simulink model "RadioReceiver_FP_clean_PIPELINED_64bit"  (R2017a)
settings: Solver=FixedStepDiscrete  StartTime=0.0  StopTime=10.0  RelTol=1e-3
InitFcn:
  | barker = comm.BarkerCode('SamplesPerFrame', 28, 'Length', 11);
  | seq = barker()+1;
  | M = 4;
  | hPSKModTrain   = comm.PSKModulator(M, ...
  |     'PhaseOffset',pi/4, ...
  |     'SymbolMapping','Binary');
  | xPreambleSeq = hPSKModTrain(seq);
  | 
  | 
  | %%%%%%%%%%%%
  | 
  | % AGC Preamble
  | reps = 5;
  | barker = comm.BarkerCode('SamplesPerFrame', 16, 'Length', 13);
  | seq = barker()+1;
  | %preamble = zeros(16*reps,1);
  | preambleFull = repmat(seq,reps,1);
  | rctFilt = comm.RaisedCosineTransmitFilter('FilterSpanInSymbols', 128,...
  | 'RolloffFactor',0.5,...
  | 'OutputSamplesPerSymbol',4);
  | preambleFullFilt = rctFilt(preambleFull);
  | 
  | %%%%%%%%%%%%
  | 
  | RadioSampleRate = 1e6;
  | %RadioSampleRate = 20e6;
  | RadioFrameLength = 1e5;
  | 
  | VibertiTracebackLength = 34+20;
  | numTrainingSamples = 250;
  | crc32Poly = [1 0 0 0 0 0 1 0 0 1 1 0 0 0 0 0 1 0 0 0 1 1 1 0 1 1 0 1 1 0 1 1 1];
  | crcDecodeLag = length(crc32Poly)-1+2;
  | 
  | %%%%%%%%%%%%
  | 
  | beta = 0.5;
  | span = 8;
  | sps = 4;
  | filterGain = 1;
  | coeff = rcosdesign(beta, span, sps, 'sqrt')*filterGain;
  | 
  | %%%%%%%%%%%%
  | 
  | samplesPerSymbol = 4;
  | maxPacketBits = 8*1500;
  | bItsPerSymbol = 2;
  | CodeRate = 2;
  | tailSymbols = 40;
  | maxPayloadSymbols = maxPacketBits*CodeRate/bItsPerSymbol+tailSymbols;
undefined symbols (not defined in the file or in its folder): j
libraries: dsphdlfiltering x20, simulink x15, dspstat3 x2, hdlsllib x2, commdigbbndpm3 x2, commsource2 x1, commcrc2 x1, commcnvcod2 x1, commseqgen3 x1, commutil2 x1
(part 2 of 2)

== system RadioReceiver_FP_clean_PIPELINED_64bit/Receiver HDL/Frame Recover/Barker Locate/Measure Phase Ambiguity1/Find Max and Set Output Shift ==
  In1 : Inport
  In2 : Inport  Port=2
  In4 : Inport  Port=3
  In5 : Inport  Port=4
  Enable : EnablePort
  Complex to Real-Imag{,1..3} (4 alike) : ComplexToRealImag  Output=Imag
  Direct Lookup Table (n-D) : LookupNDDirect  NumberOfTableDimensions=1  Table=exp(-(0:pi/2:(pi*3/2)) .* 1i).'  DiagnosticForOutOfRangeInput=Error  TableDataTypeStr=fixdt(1,16,13)
  Display : Display
  Display1 : Display
  Maximum : dspstat3/Maximum  operation=maximum  fcn=Index  indexBase=Zero  operateOver=Each column  Dimension=1  InputProcessing=Columns as channels (frame based)  reset=None  roiEnable=off  roiType=Rectangles  roiPortion=Entire ROI  roiOutput=Individual statistics for each ROI  roiFlag=off  roundingMode=Floor  overflowMode=off  accumDataTypeStr=Inherit: Same as product output  accumLastDataTypeStr=Inherit: Same as product output
  Vector Concatenate : Concatenate  NumInputs=4
  Vector Concatenate1 : Concatenate  NumInputs=4
  Out1 : Outport  InitialOutput=0
  wires:
  Direct Lookup Table (n-D)/1 -> Out1/1
  In4/1 -> Vector Concatenate1/3, Complex to Real-Imag2/1
  In2/1 -> Vector Concatenate1/2, Complex to Real-Imag1/1
  In5/1 -> Vector Concatenate1/4, Complex to Real-Imag3/1
  In1/1 -> Vector Concatenate1/1, Complex to Real-Imag/1
  Maximum/1 -> Direct Lookup Table (n-D)/1
  Vector Concatenate/1 -> Display/1, Maximum/1
  Vector Concatenate1/1 -> Display1/1
  Complex to Real-Imag1/1 -> Vector Concatenate/2
  Complex to Real-Imag3/1 -> Vector Concatenate/4
  Complex to Real-Imag2/1 -> Vector Concatenate/3
  Complex to Real-Imag/1 -> Vector Concatenate/1

== system RadioReceiver_FP_clean_PIPELINED_64bit/Receiver HDL/Frame Recover/Barker Locate/Measure Phase Ambiguity1/HDL Opt Complex FIR4 ==
  In1 : Inport
  validIn : Inport  Port=2
  Add : Sum  Inputs=+-  AccumDataTypeStr=fixdt(1,16,0)
  Complex to Real-Imag : ComplexToRealImag
  Discrete FIR Filter HDL Optimized : dsphdlfiltering/Discrete FIR Filter HDL Optimized  Numerator=real(Taps)  Sharing=off  SharingFactor=2  SimulateUsing=Code generation  roundingMode=Floor  overflowMode=off  CoefficientsDataTypeStr=Inherit: Same word length as input  CoefficientsMin=[]  CoefficientsMax=[]  OutputDataTypeStr=fixdt(1,16,0)  OutputMin=[]  OutputMax=[]  ValidInPort=on  ReadyPort=off
      settings: SourceProductName=DSP System Toolbox  SourceProductBaseCode=DS
  Discrete FIR Filter HDL Optimized1 : dsphdlfiltering/Discrete FIR Filter HDL Optimized  Numerator=imag(Taps)  Sharing=off  SharingFactor=2  SimulateUsing=Code generation  roundingMode=Floor  overflowMode=off  CoefficientsDataTypeStr=Inherit: Same word length as input  CoefficientsMin=[]  CoefficientsMax=[]  OutputDataTypeStr=fixdt(1,16,0)  OutputMin=[]  OutputMax=[]  ValidInPort=on  ReadyPort=off
      settings: SourceProductName=DSP System Toolbox  SourceProductBaseCode=DS
  Discrete FIR Filter HDL Optimized2 : dsphdlfiltering/Discrete FIR Filter HDL Optimized  Numerator=real(Taps)  Sharing=off  SharingFactor=2  SimulateUsing=Code generation  roundingMode=Floor  overflowMode=off  CoefficientsDataTypeStr=Inherit: Same word length as input  CoefficientsMin=[]  CoefficientsMax=[]  OutputDataTypeStr=fixdt(1,16,0)  OutputMin=[]  OutputMax=[]  ValidInPort=on  ReadyPort=off
      settings: SourceProductName=DSP System Toolbox  SourceProductBaseCode=DS
  Discrete FIR Filter HDL Optimized3 : dsphdlfiltering/Discrete FIR Filter HDL Optimized  Numerator=imag(Taps)  Sharing=off  SharingFactor=2  SimulateUsing=Code generation  roundingMode=Floor  overflowMode=off  CoefficientsDataTypeStr=Inherit: Same word length as input  CoefficientsMin=[]  CoefficientsMax=[]  OutputDataTypeStr=fixdt(1,16,0)  OutputMin=[]  OutputMax=[]  ValidInPort=on  ReadyPort=off
      settings: SourceProductName=DSP System Toolbox  SourceProductBaseCode=DS
  Logical Operator : Logic  Inputs=4  AllPortsSameDT=off  OutDataTypeStr=boolean
  Real-Imag to Complex : RealImagToComplex
  Subtract : Sum  OutDataTypeStr=int16
  Out1 : Outport
  validOut : Outport  Port=2
  wires:
  Discrete FIR Filter HDL Optimized/1 -> Add/1
  Logical Operator/1 -> validOut/1
  Discrete FIR Filter HDL Optimized/2 -> Logical Operator/1
  Discrete FIR Filter HDL Optimized1/2 -> Logical Operator/2
  Discrete FIR Filter HDL Optimized1/1 -> Add/2
  validIn/1 -> Discrete FIR Filter HDL Optimized3/2, Discrete FIR Filter HDL Optimized2/2, Discrete FIR Filter HDL Optimized1/2, Discrete FIR Filter HDL Optimized/2
  In1/1 -> Complex to Real-Imag/1
  Complex to Real-Imag/1 -> Discrete FIR Filter HDL Optimized3/1, Discrete FIR Filter HDL Optimized/1
  Discrete FIR Filter HDL Optimized2/2 -> Logical Operator/3
  Discrete FIR Filter HDL Optimized3/2 -> Logical Operator/4
  Complex to Real-Imag/2 -> Discrete FIR Filter HDL Optimized2/1, Discrete FIR Filter HDL Optimized1/1
  Discrete FIR Filter HDL Optimized2/1 -> Subtract/1
  Discrete FIR Filter HDL Optimized3/1 -> Subtract/2
  Real-Imag to Complex/1 -> Out1/1
  Subtract/1 -> Real-Imag to Complex/2
  Add/1 -> Real-Imag to Complex/1

== system RadioReceiver_FP_clean_PIPELINED_64bit/Receiver HDL/Frame Recover/Barker Locate/Measure Phase Ambiguity1/HDL Opt Complex FIR5 ==
  In1 : Inport
  validIn : Inport  Port=2
  Add : Sum  Inputs=+-  AccumDataTypeStr=fixdt(1,16,0)
  Complex to Real-Imag : ComplexToRealImag
  Discrete FIR Filter HDL Optimized : dsphdlfiltering/Discrete FIR Filter HDL Optimized  Numerator=real(Taps)  Sharing=off  SharingFactor=2  SimulateUsing=Code generation  roundingMode=Floor  overflowMode=off  CoefficientsDataTypeStr=Inherit: Same word length as input  CoefficientsMin=[]  CoefficientsMax=[]  OutputDataTypeStr=fixdt(1,16,0)  OutputMin=[]  OutputMax=[]  ValidInPort=on  ReadyPort=off
      settings: SourceProductName=DSP System Toolbox  SourceProductBaseCode=DS
  Discrete FIR Filter HDL Optimized1 : dsphdlfiltering/Discrete FIR Filter HDL Optimized  Numerator=imag(Taps)  Sharing=off  SharingFactor=2  SimulateUsing=Code generation  roundingMode=Floor  overflowMode=off  CoefficientsDataTypeStr=Inherit: Same word length as input  CoefficientsMin=[]  CoefficientsMax=[]  OutputDataTypeStr=fixdt(1,16,0)  OutputMin=[]  OutputMax=[]  ValidInPort=on  ReadyPort=off
      settings: SourceProductName=DSP System Toolbox  SourceProductBaseCode=DS
  Discrete FIR Filter HDL Optimized2 : dsphdlfiltering/Discrete FIR Filter HDL Optimized  Numerator=real(Taps)  Sharing=off  SharingFactor=2  SimulateUsing=Code generation  roundingMode=Floor  overflowMode=off  CoefficientsDataTypeStr=Inherit: Same word length as input  CoefficientsMin=[]  CoefficientsMax=[]  OutputDataTypeStr=fixdt(1,16,0)  OutputMin=[]  OutputMax=[]  ValidInPort=on  ReadyPort=off
      settings: SourceProductName=DSP System Toolbox  SourceProductBaseCode=DS
  Discrete FIR Filter HDL Optimized3 : dsphdlfiltering/Discrete FIR Filter HDL Optimized  Numerator=imag(Taps)  Sharing=off  SharingFactor=2  SimulateUsing=Code generation  roundingMode=Floor  overflowMode=off  CoefficientsDataTypeStr=Inherit: Same word length as input  CoefficientsMin=[]  CoefficientsMax=[]  OutputDataTypeStr=fixdt(1,16,0)  OutputMin=[]  OutputMax=[]  ValidInPort=on  ReadyPort=off
      settings: SourceProductName=DSP System Toolbox  SourceProductBaseCode=DS
  Logical Operator : Logic  Inputs=4  AllPortsSameDT=off  OutDataTypeStr=boolean
  Real-Imag to Complex : RealImagToComplex
  Subtract : Sum  OutDataTypeStr=int16
  Out1 : Outport
  validOut : Outport  Port=2
  wires:
  Discrete FIR Filter HDL Optimized/1 -> Add/1
  Logical Operator/1 -> validOut/1
  Discrete FIR Filter HDL Optimized/2 -> Logical Operator/1
  Discrete FIR Filter HDL Optimized1/2 -> Logical Operator/2
  Discrete FIR Filter HDL Optimized1/1 -> Add/2
  validIn/1 -> Discrete FIR Filter HDL Optimized3/2, Discrete FIR Filter HDL Optimized2/2, Discrete FIR Filter HDL Optimized1/2, Discrete FIR Filter HDL Optimized/2
  In1/1 -> Complex to Real-Imag/1
  Complex to Real-Imag/1 -> Discrete FIR Filter HDL Optimized3/1, Discrete FIR Filter HDL Optimized/1
  Discrete FIR Filter HDL Optimized2/2 -> Logical Operator/3
  Discrete FIR Filter HDL Optimized3/2 -> Logical Operator/4
  Complex to Real-Imag/2 -> Discrete FIR Filter HDL Optimized2/1, Discrete FIR Filter HDL Optimized1/1
  Discrete FIR Filter HDL Optimized2/1 -> Subtract/1
  Discrete FIR Filter HDL Optimized3/1 -> Subtract/2
  Real-Imag to Complex/1 -> Out1/1
  Subtract/1 -> Real-Imag to Complex/2
  Add/1 -> Real-Imag to Complex/1

== system RadioReceiver_FP_clean_PIPELINED_64bit/Receiver HDL/Frame Recover/Barker Locate/Measure Phase Ambiguity1/HDL Opt Complex FIR6 ==
  In1 : Inport
  validIn : Inport  Port=2
  Add : Sum  Inputs=+-  AccumDataTypeStr=fixdt(1,16,0)
  Complex to Real-Imag : ComplexToRealImag
  Discrete FIR Filter HDL Optimized : dsphdlfiltering/Discrete FIR Filter HDL Optimized  Numerator=real(Taps)  Sharing=off  SharingFactor=2  SimulateUsing=Code generation  roundingMode=Floor  overflowMode=off  CoefficientsDataTypeStr=Inherit: Same word length as input  CoefficientsMin=[]  CoefficientsMax=[]  OutputDataTypeStr=fixdt(1,16,0)  OutputMin=[]  OutputMax=[]  ValidInPort=on  ReadyPort=off
      settings: SourceProductName=DSP System Toolbox  SourceProductBaseCode=DS
  Discrete FIR Filter HDL Optimized1 : dsphdlfiltering/Discrete FIR Filter HDL Optimized  Numerator=imag(Taps)  Sharing=off  SharingFactor=2  SimulateUsing=Code generation  roundingMode=Floor  overflowMode=off  CoefficientsDataTypeStr=Inherit: Same word length as input  CoefficientsMin=[]  CoefficientsMax=[]  OutputDataTypeStr=fixdt(1,16,0)  OutputMin=[]  OutputMax=[]  ValidInPort=on  ReadyPort=off
      settings: SourceProductName=DSP System Toolbox  SourceProductBaseCode=DS
  Discrete FIR Filter HDL Optimized2 : dsphdlfiltering/Discrete FIR Filter HDL Optimized  Numerator=real(Taps)  Sharing=off  SharingFactor=2  SimulateUsing=Code generation  roundingMode=Floor  overflowMode=off  CoefficientsDataTypeStr=Inherit: Same word length as input  CoefficientsMin=[]  CoefficientsMax=[]  OutputDataTypeStr=fixdt(1,16,0)  OutputMin=[]  OutputMax=[]  ValidInPort=on  ReadyPort=off
      settings: SourceProductName=DSP System Toolbox  SourceProductBaseCode=DS
  Discrete FIR Filter HDL Optimized3 : dsphdlfiltering/Discrete FIR Filter HDL Optimized  Numerator=imag(Taps)  Sharing=off  SharingFactor=2  SimulateUsing=Code generation  roundingMode=Floor  overflowMode=off  CoefficientsDataTypeStr=Inherit: Same word length as input  CoefficientsMin=[]  CoefficientsMax=[]  OutputDataTypeStr=fixdt(1,16,0)  OutputMin=[]  OutputMax=[]  ValidInPort=on  ReadyPort=off
      settings: SourceProductName=DSP System Toolbox  SourceProductBaseCode=DS
  Logical Operator : Logic  Inputs=4  AllPortsSameDT=off  OutDataTypeStr=boolean
  Real-Imag to Complex : RealImagToComplex
  Subtract : Sum  OutDataTypeStr=int16
  Out1 : Outport
  validOut : Outport  Port=2
  wires:
  Discrete FIR Filter HDL Optimized/1 -> Add/1
  Logical Operator/1 -> validOut/1
  Discrete FIR Filter HDL Optimized/2 -> Logical Operator/1
  Discrete FIR Filter HDL Optimized1/2 -> Logical Operator/2
  Discrete FIR Filter HDL Optimized1/1 -> Add/2
  validIn/1 -> Discrete FIR Filter HDL Optimized3/2, Discrete FIR Filter HDL Optimized2/2, Discrete FIR Filter HDL Optimized1/2, Discrete FIR Filter HDL Optimized/2
  In1/1 -> Complex to Real-Imag/1
  Complex to Real-Imag/1 -> Discrete FIR Filter HDL Optimized3/1, Discrete FIR Filter HDL Optimized/1
  Discrete FIR Filter HDL Optimized2/2 -> Logical Operator/3
  Discrete FIR Filter HDL Optimized3/2 -> Logical Operator/4
  Complex to Real-Imag/2 -> Discrete FIR Filter HDL Optimized2/1, Discrete FIR Filter HDL Optimized1/1
  Discrete FIR Filter HDL Optimized2/1 -> Subtract/1
  Discrete FIR Filter HDL Optimized3/1 -> Subtract/2
  Real-Imag to Complex/1 -> Out1/1
  Subtract/1 -> Real-Imag to Complex/2
  Add/1 -> Real-Imag to Complex/1

== system RadioReceiver_FP_clean_PIPELINED_64bit/Receiver HDL/Frame Recover/Barker Locate/Measure Phase Ambiguity1/HDL Opt Complex FIR7 ==
  In1 : Inport
  validIn : Inport  Port=2
  Add : Sum  Inputs=+-  AccumDataTypeStr=fixdt(1,16,0)
  Complex to Real-Imag : ComplexToRealImag
  Discrete FIR Filter HDL Optimized : dsphdlfiltering/Discrete FIR Filter HDL Optimized  Numerator=real(Taps)  Sharing=off  SharingFactor=2  SimulateUsing=Code generation  roundingMode=Floor  overflowMode=off  CoefficientsDataTypeStr=Inherit: Same word length as input  CoefficientsMin=[]  CoefficientsMax=[]  OutputDataTypeStr=fixdt(1,16,0)  OutputMin=[]  OutputMax=[]  ValidInPort=on  ReadyPort=off
      settings: SourceProductName=DSP System Toolbox  SourceProductBaseCode=DS
  Discrete FIR Filter HDL Optimized1 : dsphdlfiltering/Discrete FIR Filter HDL Optimized  Numerator=imag(Taps)  Sharing=off  SharingFactor=2  SimulateUsing=Code generation  roundingMode=Floor  overflowMode=off  CoefficientsDataTypeStr=Inherit: Same word length as input  CoefficientsMin=[]  CoefficientsMax=[]  OutputDataTypeStr=fixdt(1,16,0)  OutputMin=[]  OutputMax=[]  ValidInPort=on  ReadyPort=off
      settings: SourceProductName=DSP System Toolbox  SourceProductBaseCode=DS
  Discrete FIR Filter HDL Optimized2 : dsphdlfiltering/Discrete FIR Filter HDL Optimized  Numerator=real(Taps)  Sharing=off  SharingFactor=2  SimulateUsing=Code generation  roundingMode=Floor  overflowMode=off  CoefficientsDataTypeStr=Inherit: Same word length as input  CoefficientsMin=[]  CoefficientsMax=[]  OutputDataTypeStr=fixdt(1,16,0)  OutputMin=[]  OutputMax=[]  ValidInPort=on  ReadyPort=off
      settings: SourceProductName=DSP System Toolbox  SourceProductBaseCode=DS
  Discrete FIR Filter HDL Optimized3 : dsphdlfiltering/Discrete FIR Filter HDL Optimized  Numerator=imag(Taps)  Sharing=off  SharingFactor=2  SimulateUsing=Code generation  roundingMode=Floor  overflowMode=off  CoefficientsDataTypeStr=Inherit: Same word length as input  CoefficientsMin=[]  CoefficientsMax=[]  OutputDataTypeStr=fixdt(1,16,0)  OutputMin=[]  OutputMax=[]  ValidInPort=on  ReadyPort=off
      settings: SourceProductName=DSP System Toolbox  SourceProductBaseCode=DS
  Logical Operator : Logic  Inputs=4  AllPortsSameDT=off  OutDataTypeStr=boolean
  Real-Imag to Complex : RealImagToComplex
  Subtract : Sum  OutDataTypeStr=int16
  Out1 : Outport
  validOut : Outport  Port=2
  wires:
  Discrete FIR Filter HDL Optimized/1 -> Add/1
  Logical Operator/1 -> validOut/1
  Discrete FIR Filter HDL Optimized/2 -> Logical Operator/1
  Discrete FIR Filter HDL Optimized1/2 -> Logical Operator/2
  Discrete FIR Filter HDL Optimized1/1 -> Add/2
  validIn/1 -> Discrete FIR Filter HDL Optimized3/2, Discrete FIR Filter HDL Optimized2/2, Discrete FIR Filter HDL Optimized1/2, Discrete FIR Filter HDL Optimized/2
  In1/1 -> Complex to Real-Imag/1
  Complex to Real-Imag/1 -> Discrete FIR Filter HDL Optimized3/1, Discrete FIR Filter HDL Optimized/1
  Discrete FIR Filter HDL Optimized2/2 -> Logical Operator/3
  Discrete FIR Filter HDL Optimized3/2 -> Logical Operator/4
  Complex to Real-Imag/2 -> Discrete FIR Filter HDL Optimized2/1, Discrete FIR Filter HDL Optimized1/1
  Discrete FIR Filter HDL Optimized2/1 -> Subtract/1
  Discrete FIR Filter HDL Optimized3/1 -> Subtract/2
  Real-Imag to Complex/1 -> Out1/1
  Subtract/1 -> Real-Imag to Complex/2
  Add/1 -> Real-Imag to Complex/1

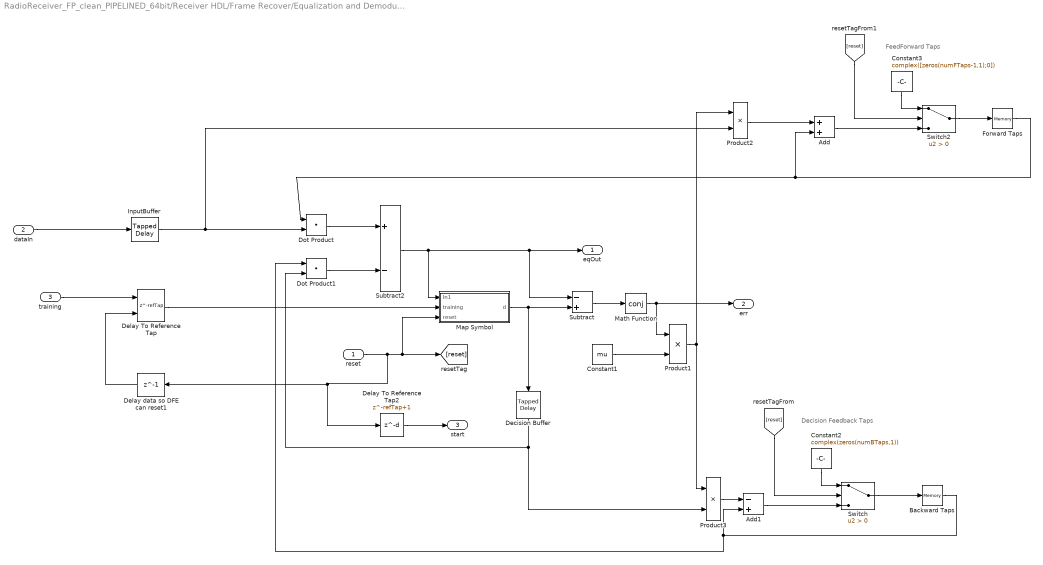
== system RadioReceiver_FP_clean_PIPELINED_64bit/Receiver HDL/Frame Recover/Equalization and Demodulation/DFE/DFE Block ==
  note: FeedForward Taps
  note: Decision Feedback Taps
  reset : Inport
  dataIn : Inport  Port=2  OutDataTypeStr=fixdt(1,16,14)  PortDimensions=1
  training : Inport  Port=3  OutDataTypeStr=fixdt(1,16,15)
  Add : Sum  OutDataTypeStr=fixdt(1,16,14)
  Add1 : Sum  Inputs=-+  OutDataTypeStr=fixdt(1,16,17)
  Backward Taps : Memory  X0=complex(zeros(numBTaps,1))  InheritSampleTime=on
  Constant1 : Constant  Value=mu  OutDataTypeStr=fixdt(0,16,20)  SampleTime=-1
  Constant2 : Constant  Value=complex(zeros(numBTaps,1))  OutDataTypeStr=fixdt(1,16,4)  SampleTime=-1
  Constant3 : Constant  Value=complex([zeros(numFTaps-1,1);0])  OutDataTypeStr=fixdt(1,16,4)  SampleTime=-1
  Decision Buffer : simulink/Discrete/Tapped Delay  vinit=0.0  samptime=-1  NumDelays=numBTaps  DelayOrder=Oldest  includeCurrent=off
  Delay To Reference Tap : Delay  DelayLength=refTap  ExternalReset=Level
      settings: InputPortMap=u0,r5
  Delay To Reference Tap2 : Delay  DelayLength=refTap+1
  Delay data so DFE can reset1 : Delay  DelayLength=1
  Dot Product : DotProduct  OutDataTypeStr=fixdt(1,16,15)  SaturateOnIntegerOverflow=on  InputSameDT=on
  Dot Product1 : DotProduct  OutDataTypeStr=fixdt(1,16,17)  SaturateOnIntegerOverflow=on  InputSameDT=on
  Forward Taps : Memory  X0=[complex(zeros(numFTaps-1,1));1]  InheritSampleTime=on
  InputBuffer : simulink/Discrete/Tapped Delay  vinit=0.0  samptime=-1  NumDelays=numFTaps  DelayOrder=Oldest  includeCurrent=off
  Map Symbol : Subsystem
  Math Function : Math  Operator=conj  RndMeth=Zero  SaturateOnIntegerOverflow=on
  Product1 : Product  OutDataTypeStr=fixdt(1,16,19)
  Product2 : Product  OutDataTypeStr=fixdt(1,16,19)
  Product3 : Product  OutDataTypeStr=fixdt(1,16,19)
  Subtract : Sum  Inputs=-+  OutDataTypeStr=fixdt(1,16,15)
  Subtract2 : Sum  Inputs=+-  OutDataTypeStr=fixdt(1,16,15)
  Switch : Switch  Criteria=u2 > Threshold  OutDataTypeStr=fixdt(1,16,15)
  Switch2 : Switch  Criteria=u2 > Threshold  OutDataTypeStr=fixdt(1,16,14)
  eqOut : Outport
  err : Outport  Port=2
  start : Outport  Port=3
  wires:
  InputBuffer/1 -> Product2/2, Dot Product/2
  Dot Product/1 -> Subtract2/1
  Dot Product1/1 -> Subtract2/2
  Subtract2/1 -> Map Symbol/1(In1), Subtract/1, eqOut/1
  Subtract/1 -> Math Function/1
  Math Function/1 -> err/1, Product1/1
  Forward Taps/1 -> Dot Product/1, Add/2
  Map Symbol/1(d) -> Subtract/2, Decision Buffer/1
  Constant1/1 -> Product1/2
  Backward Taps/1 -> Dot Product1/1, Add1/2
  Decision Buffer/1 -> Product3/2, Dot Product1/2
  Add1/1 -> Switch/3
  Switch/1 -> Backward Taps/1
  Constant2/1 -> Switch/1
  [reset] -> Switch/2
  Switch2/1 -> Forward Taps/1
  Add/1 -> Switch2/3
  Constant3/1 -> Switch2/1
  [reset] -> Switch2/2
  Product2/1 -> Add/1
  Product1/1 -> Product2/1, Product3/1
  Product3/1 -> Add1/1
  dataIn/1 -> InputBuffer/1
  Delay To Reference Tap/1 -> Map Symbol/2(training)
  reset/1 -> Delay To Reference Tap2/1, Delay data so DFE can reset1/1, [reset], Map Symbol/3(reset)
  training/1 -> Delay To Reference Tap/1
  Delay data so DFE can reset1/1 -> Delay To Reference Tap/2
  Delay To Reference Tap2/1 -> start/1

== system RadioReceiver_FP_clean_PIPELINED_64bit/Receiver HDL/Frame Recover/Equalization and Demodulation/DFE/Packeted To Unpacked ==
  In1 : Inport
  Extract Bits : simulink/Logic and Bit Operations/Extract Bits  bitsToExtract=Range of bits  numBits=8  bitIdxRange=[1]  outScalingMode=Treat bit field as an integer
      settings: SourceProductName=Simulink
  Extract Bits1 : simulink/Logic and Bit Operations/Extract Bits  bitsToExtract=Range of bits  numBits=8  bitIdxRange=[0]  outScalingMode=Treat bit field as an integer
      settings: SourceProductName=Simulink
  Vector Concatenate : Concatenate
  Out1 : Outport
  wires:
  In1/1 -> Extract Bits1/1, Extract Bits/1
  Extract Bits/1 -> Vector Concatenate/1
  Extract Bits1/1 -> Vector Concatenate/2
  Vector Concatenate/1 -> Out1/1

== system RadioReceiver_FP_clean_PIPELINED_64bit/Receiver HDL/Frame Recover/Frequency Recovery/PED For QPSK/Flip Sign ==
  In1 : Inport
  Add : Sum
  Bitwise Operator : simulink/Logic and Bit Operations/Bitwise Operator  logicop=NOT  UseBitMask=off  BitMask=bin2dec('11011001')  BitMaskRealWorld=Stored Integer
  Constant : Constant  Value=fi(0.0000306,1,16,14)  SampleTime=-1
  Out1 : Outport
  wires:
  Bitwise Operator/1 -> Add/1
  In1/1 -> Bitwise Operator/1
  Add/1 -> Out1/1
  Constant/1 -> Add/2

== system RadioReceiver_FP_clean_PIPELINED_64bit/Receiver HDL/Frame Recover/Frequency Recovery/PED For QPSK/Flip Sign1 ==
  In1 : Inport
  Add : Sum
  Bitwise Operator : simulink/Logic and Bit Operations/Bitwise Operator  logicop=NOT  UseBitMask=off  BitMask=bin2dec('11011001')  BitMaskRealWorld=Stored Integer
  Constant : Constant  Value=fi(0.0000306,1,16,14)  SampleTime=-1
  Out1 : Outport
  wires:
  Bitwise Operator/1 -> Add/1
  In1/1 -> Bitwise Operator/1
  Add/1 -> Out1/1
  Constant/1 -> Add/2

== system RadioReceiver_FP_clean_PIPELINED_64bit/Receiver HDL/Frame Recover/Gardner Reference/Gardner TED Blocks/Imag Error ==
  data : Inport
  strobe sum : Inport  Port=2
  Delay : Delay  DelayLength=1
  Product1 : Product
  Sub : Sum  Inputs=+-
  TED Buffer Update1 : Subsystem
  Out1 : Outport
  wires:
  Product1/1 -> Out1/1
  Sub/1 -> Product1/2
  data/1 -> Sub/2, Delay/1
  strobe sum/1 -> TED Buffer Update1/2(strobe sum)
  TED Buffer Update1/2(oldest) -> Sub/1
  Delay/1 -> TED Buffer Update1/1(new data)
  TED Buffer Update1/1(Middle Indx) -> Product1/1

== system RadioReceiver_FP_clean_PIPELINED_64bit/Receiver HDL/Frame Recover/Gardner Reference/Gardner TED Blocks/Real Error ==
  data : Inport
  strobe sum : Inport  Port=2
  Delay : Delay  DelayLength=1
  Product1 : Product  OutDataTypeStr=fixdt(1,16,12)
  Sub : Sum  Inputs=+-
  TED Buffer Update1 : Subsystem
  Out1 : Outport
  wires:
  Product1/1 -> Out1/1
  Sub/1 -> Product1/2
  data/1 -> Sub/2, Delay/1
  strobe sum/1 -> TED Buffer Update1/2(strobe sum)
  TED Buffer Update1/2(oldest) -> Sub/1
  Delay/1 -> TED Buffer Update1/1(new data)
  TED Buffer Update1/1(Middle Indx) -> Product1/1

== system RadioReceiver_FP_clean_PIPELINED_64bit/Receiver HDL/Frame Recover/Gardner Reference/InterpControl_Blocks1/Calculate New mu ==
  note: Good at fixd(0,16,12)
  W : Inport
  NCOCounter : Inport  Port=2
  Math Reciprocal : Math  Operator=reciprocal  OutDataTypeStr=fixdt(1,16,12)  RndMeth=Zero  SaturateOnIntegerOverflow=on
  Product : Product  OutDataTypeStr=fixdt(0,15,14)
  mu : Outport
  wires:
  Product/1 -> mu/1
  Math Reciprocal/1 -> Product/1
  NCOCounter/1 -> Product/2
  W/1 -> Math Reciprocal/1

== system RadioReceiver_FP_clean_PIPELINED_64bit/Receiver HDL/Frame Recover/Gardner Reference/InterpControl_Blocks1/Mod 1 ==
  In1 : Inport
  Add : Sum
  Compare To Constant : simulink/Logic and Bit Operations/Compare To Constant  relop=<  const=1  OutDataTypeStr=boolean
  Compare To Constant1 : simulink/Logic and Bit Operations/Compare To Constant  relop=>=  const=0  OutDataTypeStr=boolean
  Constant : Constant  OutDataTypeStr=fixdt(0,1,0)  SampleTime=-1
  Constant1 : Constant  OutDataTypeStr=fixdt(0,1,0)  SampleTime=-1
  Logical Operator : Logic  AllPortsSameDT=off  OutDataTypeStr=boolean
  Subtract : Sum  Inputs=+-
  Switch : Switch  Criteria=u2 > Threshold
  Switch1 : Switch
  Out1 : Outport
  wires:
  Switch/1 -> Out1/1
  Constant/1 -> Subtract/2
  Constant1/1 -> Add/2
  Switch1/1 -> Switch/3
  Subtract/1 -> Switch1/1
  Add/1 -> Switch1/3
  In1/1 -> Switch1/2, Compare To Constant1/1, Compare To Constant/1, Switch/1, Add/1, Subtract/1
  Compare To Constant1/1 -> Logical Operator/1
  Compare To Constant/1 -> Logical Operator/2
  Logical Operator/1 -> Switch/2

== system RadioReceiver_FP_clean_PIPELINED_64bit/Receiver HDL/Frame Recover/Equalization and Demodulation/DFE/DFE Block/Map Symbol ==
  In1 : Inport  OutDataTypeStr=fixdt(1,16,15)
  training : Inport  Port=2  OutDataTypeStr=fixdt(1,16,15)
  reset : Inport  Port=3
  Decision Directed : Subsystem
  Delay : Delay  DelayLength=1
  HDL Counter : hdlsllib/HDL Operations/HDL Counter  CountType=Count limited  CountInit=0  CountStep=1  CountMax=2^18  CountFromType=Initial value  CountFrom=0  CountResetPort=on  CountLoadPort=off  CountEnbPort=off  CountDirPort=off  CountDataType=Unsigned  CountWordLen=32  CountFracLen=0  CountSampTime=1
      settings: SourceProductName=HDL Coder  SourceProductBaseCode=HD
  Switch : Switch  Criteria=u2 > Threshold  Threshold=numTrainingSamples  OutDataTypeStr=fixdt(1,16,15)
  d : Outport
  wires:
  In1/1 -> Decision Directed/1(eqOut)
  Switch/1 -> d/1
  reset/1 -> HDL Counter/1
  Decision Directed/1(decision) -> Switch/1
  training/1 -> Delay/1
  Delay/1 -> Switch/3
  HDL Counter/1 -> Switch/2

== system RadioReceiver_FP_clean_PIPELINED_64bit/Receiver HDL/Frame Recover/Gardner Reference/Gardner TED Blocks/Imag Error/TED Buffer Update1 ==
  new data : Inport
  strobe sum : Inport  Port=2
  Delay{,1..3} (4 alike) : Delay  DelayLength=1
  Multiport Switch{,1..3} (4 alike) : MultiPortSwitch  DataPortOrder=Zero-based contiguous  DataPortIndices={0,1,[2,3]}
  Zero bit : Constant  Value=0  OutDataTypeStr=fixdt(1,16,13)  SampleTime=1/RadioSampleRate
  Middle Indx : Outport
  oldest : Outport  Port=2
  wires:
  strobe sum/1 -> Multiport Switch3/1, Multiport Switch2/1, Multiport Switch1/1, Multiport Switch/1
  Delay/1 -> Multiport Switch/2
  Delay1/1 -> Multiport Switch/3, Multiport Switch1/2
  Delay2/1 -> Multiport Switch/4, Multiport Switch1/3, Multiport Switch2/2
  new data/1 -> Multiport Switch3/4, Multiport Switch3/3
  Zero bit/1 -> Multiport Switch2/4
  Delay3/1 -> Multiport Switch1/4, Multiport Switch2/3, Multiport Switch3/2
  Multiport Switch1/1 -> Delay1/1
  Multiport Switch2/1 -> Middle Indx/1, Delay2/1
  Multiport Switch3/1 -> Delay3/1
  Multiport Switch/1 -> Delay/1, oldest/1

== system RadioReceiver_FP_clean_PIPELINED_64bit/Receiver HDL/Frame Recover/Gardner Reference/Gardner TED Blocks/Real Error/TED Buffer Update1 ==
  new data : Inport
  strobe sum : Inport  Port=2
  Delay{,1..3} (4 alike) : Delay  DelayLength=1
  Multiport Switch{,1..3} (4 alike) : MultiPortSwitch  DataPortOrder=Zero-based contiguous  DataPortIndices={0,1,[2,3]}
  Zero bit : Constant  Value=0  OutDataTypeStr=fixdt(1,16,13)  SampleTime=1/RadioSampleRate
  Middle Indx : Outport
  oldest : Outport  Port=2
  wires:
  strobe sum/1 -> Multiport Switch3/1, Multiport Switch2/1, Multiport Switch1/1, Multiport Switch/1
  Delay/1 -> Multiport Switch/2
  Delay1/1 -> Multiport Switch/3, Multiport Switch1/2
  Delay2/1 -> Multiport Switch/4, Multiport Switch1/3, Multiport Switch2/2
  new data/1 -> Multiport Switch3/4, Multiport Switch3/3
  Zero bit/1 -> Multiport Switch2/4
  Delay3/1 -> Multiport Switch1/4, Multiport Switch2/3, Multiport Switch3/2
  Multiport Switch1/1 -> Delay1/1
  Multiport Switch2/1 -> Middle Indx/1, Delay2/1
  Multiport Switch3/1 -> Delay3/1
  Multiport Switch/1 -> Delay/1, oldest/1

== system RadioReceiver_FP_clean_PIPELINED_64bit/Receiver HDL/Frame Recover/Equalization and Demodulation/DFE/DFE Block/Map Symbol/Decision Directed ==
  eqOut : Inport  OutDataTypeStr=fixdt(1,16,15)
  Compare To Zero : simulink/Logic and Bit Operations/Compare To Zero  relop=>=  OutDataTypeStr=boolean
  Compare To Zero1 : simulink/Logic and Bit Operations/Compare To Zero  relop=>=  OutDataTypeStr=boolean
  Complex to Real-Imag : ComplexToRealImag
  QPSK Decisions : LookupNDDirect  Table=[-0.7071 - 0.7071i, -0.7071 + 0.7071i; 0.7071 - 0.7071i, 0.7071 + 0.7071i]  DiagnosticForOutOfRangeInput=Error  TableDataTypeStr=fixdt(1,16,15)
  decision : Outport
  wires:
  eqOut/1 -> Complex to Real-Imag/1
  Complex to Real-Imag/1 -> Compare To Zero/1
  Complex to Real-Imag/2 -> Compare To Zero1/1
  Compare To Zero/1 -> QPSK Decisions/1
  Compare To Zero1/1 -> QPSK Decisions/2
  QPSK Decisions/1 -> decision/1

== matlab function RadioReceiver_FP_clean_PIPELINED_64bit/Receiver HDL/CRC Check and DMA Pack/CRC Check ES/Debug CRC input ==
  data: u input; enable input; endFlag input; startFlag input
function fcn(u, enable,endFlag,startFlag)

persistent buffer crc count

if isempty(buffer)
   buffer = false(1700,1); 
    crc = comm.CRCDetector('Polynomial','z^32 + z^26 + z^23 + z^22 + z^16 + z^12 + z^11 + z^10 + z^8 + z^7 + z^5 + z^4 + z^2 + z + 1');
    count = 1;
end

if enable
    %buffer = [buffer(2:end);u];
    if startFlag
        count = 1;
    elseif count>1700-1
        count = 1;
    else
        count = count + 1;
    end
    buffer(count) = u;
    
    if endFlag
        disp(count)
        k = buffer(1:1632);
        [~,e] = crc(k);
        if e
            disp('Error');
        else
            disp('Pass');
        end
    end
    
end

== matlab function RadioReceiver_FP_clean_PIPELINED_64bit/Receiver HDL/Frame Recover/Enable Equalizer and Packet Decode (Latch) ==
  data: start input; enable output; validIn input
function enable = Counter(start,validIn)

persistent count maxCount lastEOF

if isempty(count)
    count = uint32(0);
    maxCount = uint32(2^16); % Largest possible packet length
    lastEOF = false;
end

eof = false;

if validIn
    % Got a barker preamble start allowing data into equalizer
    if start
        count = maxCount;
    end
    
    % Check on change from true to false
    if lastEOF && ~eof
        %     fprintf('Frame end reached\n');
        count = uint32(0);
    end
    lastEOF = eof;
    
    % Past end of max frame size
    if count>0
        count = count - uint32(1);
    end
    
    % Enable downstream
    enable = count>uint32(0);
else
    enable = false;
end

== matlab function RadioReceiver_FP_clean_PIPELINED_64bit/Check Receiver/DMA Capture ==
  data: bytes input; validOut input; sync input; payloadLen input
function fcn(bytes, validOut, sync, payloadLen)

persistent frameBuffer byteCounter fullPayloadBits

bitsInPack = 64;

if isempty(frameBuffer)
    maxFrameBits = (2^16)*8;
    frameBuffer = false(maxFrameBits,1);
    byteCounter = 0;
    fullPayloadBits = uint16(0);
end

if validOut
    if sync
        byteCounter = bitsInPack;
        frameBuffer(1:byteCounter) = bitget(bytes,1:bitsInPack);
        fullPayloadBits = uint16(payloadLen*8);
        
    elseif byteCounter<fullPayloadBits
        frameBuffer(byteCounter+1:byteCounter+bitsInPack) = bitget(bytes,1:bitsInPack);
        byteCounter = byteCounter + bitsInPack;
    else
        if bytes>0
            disp('CRC Error (Outside)');
        else
            disp('Frame passed CRC (Outside)');
        end
    end
end

== matlab function RadioReceiver_FP_clean_PIPELINED_64bit/Receiver HDL/CRC Check and DMA Pack/CRC Check ES/Check CRC Result (DEBUG) ==
  data: bits input; start input; done input; valid input; err input
function fcn(bits, start, done, valid, err)

persistent buffer

if isempty(buffer)
    buffer = fi(false(1032,1),0,1,0);
end

buffer = [buffer(2:end);bits];

if done && valid
    if err
        fprintf('CRC Error (HDL CRC)\n');
    else
        fprintf('CRC Passed (HDL CRC)\n');
    end
end
if err % Flag if any error every occurs, if it occurs alone it means given crc is not long enough
    fprintf('CRC Error Type 2 (HDL CRC)\n');
end

== matlab function RadioReceiver_FP_clean_PIPELINED_64bit/Receiver HDL/Frame Recover/Equalization and Demodulation/DFE/Equalizer ==
  data: trigger input; eqOut output; data input; trainingSymbol input
function eqOut  = dfe(trigger,data,trainingSymbol)

persistent inputBuffer decisionBuffer forwardTaps backwardTaps processedSamples


%% Constants
WL = uint8(16); FL = uint8(14);
F = fimath('SumMode','SpecifyPrecision','SumWordLength',WL,...
    'SumFractionLength',FL);
% Initial delay guess
channelDelay = uint8(0);
% Equalizer settings
mu = fi(0.05,0,10,12);
nFTaps = uint8(11);
nBTaps = uint8(3);
numTrainingSymbols = uint16(250);
resetTaps = fi([complex(zeros(nFTaps-1,1));1],1,WL,FL,F);

%% Async
if isempty(inputBuffer)
    % Set Precisions
    inputBuffer = fi(complex(zeros(nFTaps,1)),1,WL,FL,F);
    decisionBuffer = fi(complex(zeros(nBTaps,1)),1,WL,FL,F);
    forwardTaps = fi(complex(zeros(nFTaps,1)),1,WL,FL,F);
    backwardTaps = fi(complex(zeros(nBTaps,1)),1,WL,FL,F);
    processedSamples = numTrainingSymbols + uint16(1); % Force to DD mode to start
end

%% Reset
if trigger
    processedSamples = uint16(0);
    % Reset taps
    %forwardTaps = fi(complex(zeros(nFTaps,1)),1,WL,FL,F);
    %forwardTaps(nFTaps-channelDelay) = fi(1,1,WL,FL); % Favor specific delay (causes equalizer to converge faster)
    forwardTaps = resetTaps;
    backwardTaps = fi(complex(zeros(nBTaps,1)),1,WL,FL,F);
    % Default output
    eqOut = fi(0,1,WL,FL,F);
else
    %% Equalizer
    % Add data to buffer
    inputBuffer = [inputBuffer(2:end);data];
    
    % Apply equalizer
    eqOut = forwardTaps'*inputBuffer - backwardTaps'*decisionBuffer;
    
    % Determine error
    if (processedSamples<numTrainingSymbols) && (processedSamples>=channelDelay)
        processedSamples = processedSamples + 1;
        d = trainingSymbol;
    else % Decision directed
        % Find closest symbol
        r = real(eqOut)>0; i = imag(eqOut)>0;
        if r
            if i
                d = fi(0.7071 + 0.7071i,1,WL,FL);
            else
                d = fi(0.7071 - 0.7071i,1,WL,FL);
            end
        else
            if i
                d = fi(-0.7071 + 0.7071i,1,WL,FL);
            else
                d = fi(-0.7071 - 0.7071i,1,WL,FL);
            end
        end
    end
    ec = conj(d - eqOut);
    
    % Update taps
    forwardTaps = forwardTaps + mu*ec*inputBuffer;
    backwardTaps = backwardTaps - mu*ec*decisionBuffer;
    
    % Update decision buffer
    db = fi(d,1,WL,FL,F);
    decisionBuffer = [db; decisionBuffer(1:end-1)];
    
end



end

== matlab function RadioReceiver_FP_clean_PIPELINED_64bit/Receiver HDL/Frame Recover/Frequency Recovery/PED ==
  data: In input; e output
function e  = PED(In)

OP2 = real(In);
OP1 = imag(In);

Real = OP2;
Imag = OP1;

if (bitget(Real,16)==true) % real component is negative
    OP1 = fi(-Imag,1,16,13);
end
if (bitget(Imag,16)==true) % imaginary component is negative
    OP2 = fi(-Real,1,16,13);
end

e= fi(OP1-OP2,1,16,10);

%e = sign(real(In)).*imag(In) - sign(imag(In)).*real(In);

== matlab function RadioReceiver_FP_clean_PIPELINED_64bit/Receiver HDL/CRC Check and DMA Pack/DMA Interface/Bit Packer ==
  data: bitIn input; byteOut output; startIn input; endIn input; err input; validIn input; validOut output; startOut output
function [byteOut,validOut,startOut] = BitPacker(bitIn, startIn, endIn, err, validIn)

% This block will pack bits into bytes with start boundaries


% Constants
bits2Pack = uint8(64); % byteReg must contain this many bits
% NOTE: Frames but be a multiple of bits2Pack or bits will be trimmed from
% end

persistent byteReg byteIndx setStartFlag

if isempty(byteIndx)
    byteReg  = fi(0,0,64,0);
    byteIndx = uint8(1);
    setStartFlag = false;
end

if validIn
    if startIn % Reset
        bitset(byteReg,1,bitIn);
        byteIndx = uint8(2);
        validOut = false;
        setStartFlag = true;
        startOut = false;
    else
        byteReg = bitset(byteReg,byteIndx,bitIn);
        if byteIndx >= bits2Pack
            byteIndx = uint8(1);
            validOut = true;
            startOut = setStartFlag;
            setStartFlag = false;
        else
            byteIndx = byteIndx + uint8(1);
            validOut = false;
            startOut = false;
        end
    end
elseif endIn % Append error bit to last byte
    byteReg = fi(err,0,64,0);
    validOut = true;
    startOut = false;
else
    validOut = false;
    startOut = false;
end

byteOut = byteReg;

== matlab function RadioReceiver_FP_clean_PIPELINED_64bit/Receiver HDL/Frame Recover/Frequency Recovery/Loop Filter/Flip Sign ==
  data: u input; y output
function y = fcn(u)

WL = 25;
FP = 20;

% Flip sign x = (~y) + 1
u8 = bitcmp(int8(u));
y = fi(u8+int8(1),1,WL,FP);

== matlab function RadioReceiver_FP_clean_PIPELINED_64bit/Receiver HDL/Frame Recover/Equalization and Demodulation/2 Bit Descrambler/MATLAB Function ==
  data: bits input; bufferA output; reset input; bufferB output
function [bufferA, bufferB] = BufferSelect(bits,reset)

persistent buffer

% Constants
initBuffer = logical([0 1 0 0 0 1 0]);

% Async
if isempty(buffer)
    buffer = initBuffer;
end

% Reset/Sync
if reset
    bufferA = initBuffer;
    bufferB = [bits(1),initBuffer(1:end-1)];
    buffer = [bits(2),bits(1),initBuffer(1:end-2)];
else
    bufferA = buffer;
    bufferB = [bits(1),buffer(1:end-1)];
    buffer = [bits(2),bits(1),buffer(1:end-2)];    
end

== matlab function RadioReceiver_FP_clean_PIPELINED_64bit/Receiver HDL/CRC Check and DMA Pack/overdrive ==
  data: validIn input; enableCRC output; endIn input
function enableCRC = fcn(validIn,endIn)

% This block drives the enabled subsystem and additional step so the
% outputs do not stay high but reset.  All signals are reset since the
% driving valid signal is false

persistent gotEndOut

if isempty(gotEndOut)
    gotEndOut = false;
end
    
if validIn
    enableCRC = true;
    gotEndOut = false;
else
    if endIn
        gotEndOut = true;
        enableCRC = true;
    elseif gotEndOut
        enableCRC = true;
    else
        enableCRC = false;
    end
end

== matlab function RadioReceiver_FP_clean_PIPELINED_64bit/Receiver HDL/Descramble and Decode/Find packet tail and check CRC (DEBUG ONLY) ==
  data: u input; enable output; crcCase output
function [enable, crcCase]=findTail(u)

persistent tailBits buffer counter head

if isempty(tailBits)
   tailBits = repmat(uint8([1 0 1 1 0 0 1 1 1 1].'),4,1);
   buffer = uint8(zeros(size(tailBits)));
    counter = 0;
    head = uint8(ones(16,1));
end

%buffer = [u; buffer(1:end-1)];
buffer = [buffer(2:end); u];
counter = counter + 2; % Coded bit counter

% Check for tail sequence
found = 0;
if isequal(buffer,tailBits)
   fprintf('Found tail after %d coded bits\n',int64(counter));
   counter = 0;
   found = 1;
end

%% CHECK CRC
persistent crc buffer2
CRCLen = 32;
nPayLoad = 8*200;
nTB = length(tailBits);

if isempty(crc)
    crc = comm.CRCDetector('Polynomial','z^32 + z^26 + z^23 + z^22 + z^16 + z^12 + z^11 + z^10 + z^8 + z^7 + z^5 + z^4 + z^2 + z + 1');
    buffer2 = false(CRCLen+nPayLoad+nTB,1);%false(10532+40,1);
end

crcCase = 0;
enable = false;

buffer2 = [buffer2(2:end); u>0];
%if isequal(head, buffer2(end-15:end))
%   fprintf('Head FOUND %d\n',int64(counter));
%end
if found>0
    NoTailBits = buffer2(1:end-nTB);
    PayloadWithCRC= NoTailBits(end-nPayLoad-CRCLen+1:end);
    enable = true;
    [~,e] = crc(PayloadWithCRC);
    if ~e
        crcCase = 1;
        fprintf('Packet CRC Passed\n');
    else
        crcCase = 0;
        fprintf('Packet CRC Failed\n');
    end
    
end

== matlab function RadioReceiver_FP_clean_PIPELINED_64bit/Receiver HDL/Frame Recover/Equalization and Demodulation/Header Controller ==
  data: headerStart input; enableDownstream output; packetLenBitsOut output; data input; resetViterbi output; crcStart output
function [enableDownstream,packetLenBitsOut,resetViterbi,crcStart] = EvalHeader(headerStart, data)

persistent counter sum1 sum2 packetLenBits lastMode savedPacketLenBits

% The header contains 16 bits, but each bit is duplicated to make checking
% easier

% Note this block works on symbols (2bits) but 1 symbol -> 1 decoded bit

% PacketLength = (Data+CRC+40(TB)+68)/CodeRate

% NOTE TAIL BITS HERE ARE REALLY USED TO DEAL WITH VITERBI LAG SO:
% TailBitsWithLagPadding > TracebackLength

%% Constants
numHeaderBits = uint8(16); % Header is this many bits
powersOfTwo = uint32([1 2 4 8 16 32 64 128 256 512 1024 2048 4096 8192 16384 32768]);
%TracebackLength = uint32(34)+uint32(20);
%CRCLen = uint32(32);
CodeRateINV = uint32(2);%1/CodeRate;
TailBitsWithLagPadding = uint32(uint32(40)+34*2+1);
% Flag when CRC porition of packet starts relative to header
%crcSignalStartLocation = uint32((TailBitsWithLagPadding+CRCLen)*CodeRateINV); % Must be even
crcSignalStartLocation = uint32((TailBitsWithLagPadding)*CodeRateINV); % Must be even

% Async
if isempty(counter)
    packetLenBits = uint32(0);
    sum1 = uint32(0);
    sum2 = uint32(0);
    counter = uint8(numHeaderBits);
    lastMode = uint8(3);
    savedPacketLenBits = uint16(0);
end

%% Sync
% Got a header now enable certain mode
if headerStart
    mode = uint8(0);
else
    mode = lastMode;
end

switch mode
    %% Reset on preamble flag and setup for header processing
    case uint8(0)
        crcStart = false;
        resetViterbi = false;
        enableDownstream = false;
        sum1 = uint32(0);
        sum2 = uint32(0);
        counter = uint8(1);
        lastMode = uint8(1); % Go to next state
        packetLenBitsOut = uint16(0);
        
    %% Process header
    case 1 
        crcStart = false;
        enableDownstream = false; %%%%%%%%%%% CHECK!
        
        % Convert header bits (bit by bit)
        if data(1)
            sum1 = sum1 + powersOfTwo(counter);
        end
        if data(2)
            sum2 = sum2 + powersOfTwo(counter);
        end
        counter = counter + uint8(1);
        
        if counter>numHeaderBits
            % Check header
            if sum1~=sum2 % Fail
                packetLenBits = uint32(0);
                lastMode = uint8(3);
                resetViterbi = false;
                packetLenBitsOut = uint16(0);
                savedPacketLenBits = uint16(0);
%                 fprintf('Header Check failed (possible false detection)\n');
%                 fprintf('sum1: %d\n',int32(sum1));
%                 fprintf('sum2: %d\n',int32(sum2));
            else % Pass
                % Saved header info and trigger downstream
                packetLenBits = uint32(sum1);
                lastMode = uint8(2);
                resetViterbi = true;
                packetLenBitsOut = uint16(sum1-crcSignalStartLocation);
                savedPacketLenBits = uint16(sum1-crcSignalStartLocation);
%                 fprintf('Header Found | Packet is %d bits long\n',int32(sum1));            
            end
        else
            packetLenBitsOut = uint16(0);
            resetViterbi = false;
        end
        
    %% Decrement sample counter
    case 2 
        resetViterbi = false;
        crcStart = (packetLenBits==crcSignalStartLocation);
        if packetLenBits>uint32(0)
            enableDownstream = true;
            packetLenBits = packetLenBits - uint32(2); % We get 2 bits each call
            packetLenBitsOut = savedPacketLenBits;
        else
            enableDownstream = false;
            lastMode = uint8(3);
            packetLenBitsOut = uint16(0); %Reset
            savedPacketLenBits = uint16(0);%Reset
        end
            
    %% Not processing anything
    otherwise % mode>2
        crcStart = false;
        resetViterbi = false;
        enableDownstream = false;
        packetLenBitsOut = uint16(0);
end

%%

% % Set default flags, which may change
% resetViterbi = false;
% crcStart = false;
% 
% % Reset when preamble found (barker sequence)
% if headerStart
%     sum1 = uint32(0);
%     sum2 = uint32(0);
%     counter = uint32(1);
% end
% 
% % Send data downstream to
% enableDownstream = packetLenBits>uint32(0);
% 
% % Flag when we are in CRC section of packet
% % Enable signal will relate to first bit of CRC portion of packet
% if packetLenBits==crcSignalStartLocation
%     crcStart = true;
% end
% 
% % Decrement packet length counter
% if enableDownstream
%     packetLenBits = packetLenBits - uint32(2); % Get 2 bits each call
% end
% 
% % Process header
% if counter<=headerBits
%     % Convert header bits (bit by bit)
%     if data(1)
%         sum1 = sum1 + powersOfTwo(counter);
%     end
%     if data(2)
%         sum2 = sum2 + powersOfTwo(counter);
%     end
%     counter = counter + uint32(1);
%     
%     if counter>headerBits
%         % Check header
%         if sum1~=sum2
%             packetLenBits = uint32(0);
%             enableDownstream = false;
%             fprintf('Header Check failed (possible false detection)\n');
%         else
%             % Saved header info and trigger downstream
%             packetLenBits = uint32(sum1);
%             fprintf('Header Found | Packet is %d bits long\n',int32(sum1));
%             resetViterbi = true;
%             enableDownstream = true;
%         end
%     end
%     
% end

== matlab function RadioReceiver_FP_clean_PIPELINED_64bit/Receiver HDL/Frame Recover/Equalization and Demodulation/MATLAB Function ==
  data: d1 input; d2 input
function fcn(d1, d2)


if isequal(d1,d2) && ~isequal(d1,zeros(16,1))
    disp('Equal');
end

== matlab function RadioReceiver_FP_clean_PIPELINED_64bit/Receiver HDL/Frame Recover/Equalization and Demodulation/MATLAB Function1 ==
  data: start input; qpsk input; bits input
function fcn(start,qpsk, bits)

persistent buffer buffer2 HeaderDataPad count

if isempty(buffer)
    buffer = complex(zeros(16,1));
    buffer2 = false(32,1);
    
    HeaderLen = 16; % Bits
    %PayloadCodedLen = (length(frame)+0)/rate;
    PayloadCodedLen = 3480;
    HeaderData = bitget(PayloadCodedLen,1:HeaderLen).';
    
    % Repeatatively encode bits
    HeaderDataPad = reshape([HeaderData HeaderData].',1,HeaderLen*2).';
    count = 0;
end

if start
    disp('start');
    count = 0;
end
count = count + 1;
buffer = [buffer(2:end);double(qpsk)];
buffer2 = [buffer2(3:end);bits(:)];
if isequal(HeaderDataPad,buffer2)
    disp('Found');
end
